simulink model "SHIP_DOWN_PT2000_matlab_2017"  (R2018b)
settings: Solver=ode8  StartTime=0.0  StopTime=2.5  RelTol=1e-3
undefined symbols (not defined in the file): Cout_c, Cout_r, Cvh_c, Cvh_r, dellay_f1, dellay_f2, dellay_f3, dellay_f4, dellay_f5, dellay_f6, DiscIntNeverNeededParam, f, L1_l, L1_r, Lvh_l, Lvh_r, R_out, Uout, Uvh
libraries: powerlib x92, simulink x18, simulink_extras x18, powerlib_meascontrol x13
(part 1 of 2)
settings Model: Creator=Anton  LastModifiedBy=VID Company
settings SFSimCC: SimUseLocalCustomCode=off
settings RTWCC: RTWUseLocalCustomCode=off
settings CodeAppCC: StateflowObjectComments=on
settings SimscapeCC: SimscapeNormalizeSystem=off

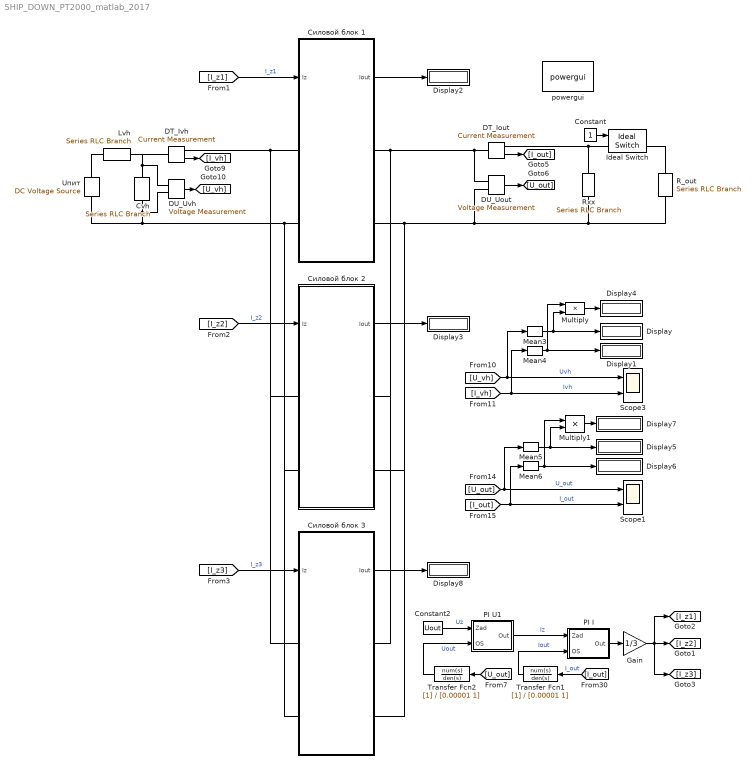
== system SHIP_DOWN_PT2000_matlab_2017 ==
  Constant : Constant
  Constant2 : Constant  Value=Uout
  Cvh : powerlib/Elements/Series RLC Branch  LConnTagsString=__new0  RConnTagsString=__new0  BranchType=RC  Resistance=Cvh_r  Inductance=1e-3  SetiL0=off  InitialCurrent=0  Capacitance=Cvh_c  Setx0=on  InitialVoltage=Uvh  Measurements=Branch voltage
      settings: SourceProductName=Simscape Electrical
  DT_Iout : powerlib/Measurements/Current Measurement  PhasorSimulation=off  OutputType=Complex  PSBequivalent=0
      settings: SourceProductName=Simscape Electrical
  DT_Ivh : powerlib/Measurements/Current Measurement  PhasorSimulation=off  OutputType=Complex  PSBequivalent=0
      settings: SourceProductName=Simscape Electrical
  DU_Uout : powerlib/Measurements/Voltage Measurement  PhasorSimulation=off  OutputType=Complex  PSBequivalent=0
      settings: SourceProductName=Simscape Electrical
  DU_Uvh : powerlib/Measurements/Voltage Measurement  PhasorSimulation=off  OutputType=Complex  PSBequivalent=0
      settings: SourceProductName=Simscape Electrical
  Display{,1..8} (9 alike) : Display
  Gain : Gain  Gain=1/3
  Ideal Switch : powerlib/Power Electronics/Ideal Switch  Ron=0.001  Lon=0  IC=0  Rs=1e5  Cs=inf  Measurements=on
  Lvh : powerlib/Elements/Series RLC Branch  LConnTagsString=__new0  RConnTagsString=__new0  BranchType=RL  Resistance=Lvh_r  Inductance=Lvh_l  SetiL0=off  InitialCurrent=0  Capacitance=1e-6  Setx0=off  InitialVoltage=0  Measurements=None
      settings: SourceProductName=Simscape Electrical
  Mean{3..6} (4 alike) : powerlib_meascontrol/Measurements/Mean  Freq=1000  Vinit=0  Ts=0
  Multiply : Product
  Multiply1 : Product
  PI I : Subsystem
  PI U1 : Subsystem
  R_out : powerlib/Elements/Series RLC Branch  LConnTagsString=__new0  RConnTagsString=__new0  BranchType=R  Resistance=R_out  Inductance=1e-3  SetiL0=off  InitialCurrent=0  Capacitance=1e-6  Setx0=off  InitialVoltage=0  Measurements=None
      settings: SourceProductName=Simscape Electrical
  Rxx : powerlib/Elements/Series RLC Branch  LConnTagsString=__new0  RConnTagsString=__new0  BranchType=R  Resistance=200  Inductance=1e-3  SetiL0=off  InitialCurrent=0  Capacitance=Cout_c  Setx0=on  InitialVoltage=0  Measurements=Branch voltage
      settings: SourceProductName=Simscape Electrical
  Scope1 : Scope  NumInputPorts=2
  Scope3 : Scope  NumInputPorts=2
  Transfer Fcn1 : TransferFcn  Denominator=[0.00001 1]
  Transfer Fcn2 : TransferFcn  Denominator=[0.00001 1]
  Uпит : powerlib/Electrical Sources/DC Voltage Source  Amplitude=Uvh  Measurements=None
      settings: SourceProductName=Simscape Electrical
  powergui : powerlib/powergui  Priority=1  SimulationMode=Discrete  SampleTime=1e-6  frequency=60  Iterations=50  frequencyindice=0  Pbase=100e6  ErrMax=1e-4  UnitsV=kV  UnitsW=MW  buscounter=0  FunctionMessages=off  echomessages=off  EnableUseOfTLC=off  CurrentSourceSwitches=off  DisableSnubberDevices=off  DisableRonSwitches=off  DisableVfSwitches=off  DisplayEquations=off  SolverType=Tustin/Backward Euler (TBE)  Interpol=off  ExternalGateDelay=off  methode=off  Ts=100  x0status=blocks  SPID=off  SwTol=0  HookPort=off  RestoreLinks=warning  ResistiveCurrentMeasurement=off  Frange=[0:2:500]  Ylog=off  Xlog=on  ShowGrid=off  save=off  variable=ZData  structure=0  ZoomFFT=off  StartTime=0.0  cycles=1  DisplayStyle=1  fundamental=60  FreqAxis=off  MaxFrequency=1000  frequencyindicesteady=1  RmsSteady=1  display=off
  Силовой блок 1 : Subsystem
  Силовой блок 2 : Subsystem
  Силовой блок 3 : Subsystem
  wires:
  Transfer Fcn2/1 -> PI U1/2(OS)  "Uout"
  PI U1/1(Out) -> PI I/1(Zad)  "Iz"
  Constant2/1 -> PI U1/1(Zad)  "Uz"
  DT_Iout/1 -> [I_out]
  DU_Uout/1 -> [U_out]
  [U_out] -> Transfer Fcn2/1
  DT_Ivh/1 -> [I_vh]
  DU_Uvh/1 -> [U_vh]
  [I_vh] -> Scope3/2, Mean4/1  "Ivh"
  [U_vh] -> Mean3/1, Scope3/1  "Uvh"
  Mean3/1 -> Display/1, Multiply/2
  Mean4/1 -> Display1/1, Multiply/1
  Multiply/1 -> Display4/1
  [U_out] -> Mean5/1, Scope1/1  "U_out"
  [I_out] -> Mean6/1, Scope1/2  "I_out"
  [I_out] -> Transfer Fcn1/1  "I_out"
  Transfer Fcn1/1 -> PI I/2(OS)  "Iout"
  PI I/1(Out) -> Gain/1
  Constant/1 -> Ideal Switch/1
  Gain/1 -> [I_z3], [I_z1], [I_z2]
  Силовой блок 1/1(Iout) -> Display2/1
  [I_z1] -> Силовой блок 1/1(Iz)  "I_z1"
  Multiply1/1 -> Display7/1
  Mean6/1 -> Display6/1, Multiply1/1
  Mean5/1 -> Display5/1, Multiply1/2
  [I_z2] -> Силовой блок 2/1(Iz)  "I_z2"
  [I_z3] -> Силовой блок 3/1(Iz)  "I_z3"
  Силовой блок 2/1(Iout) -> Display3/1
  Силовой блок 3/1(Iout) -> Display8/1
  connections:
  Cvh/RConn1 -- Силовой блок 3/LConn2 -- Силовой блок 2/LConn2 -- Силовой блок 1/LConn2 -- Uпит/LConn1 -- DU_Uvh/LConn2
  Lvh/LConn1 -- Uпит/RConn1
  Ideal Switch/RConn1 -- R_out/LConn1
  Силовой блок 3/RConn1 -- Силовой блок 2/RConn1 -- DU_Uout/LConn1 -- DT_Iout/LConn1 -- Силовой блок 1/RConn1
  DU_Uvh/LConn1 -- DT_Ivh/LConn1 -- Lvh/RConn1 -- Cvh/LConn1
  Rxx/RConn1 -- R_out/RConn1 -- Силовой блок 3/RConn2 -- Силовой блок 2/RConn2 -- Силовой блок 1/RConn2 -- DU_Uout/LConn2
  DT_Ivh/RConn1 -- Силовой блок 3/LConn1 -- Силовой блок 2/LConn1 -- Силовой блок 1/LConn1
  Ideal Switch/LConn1 -- DT_Iout/RConn1 -- Rxx/LConn1

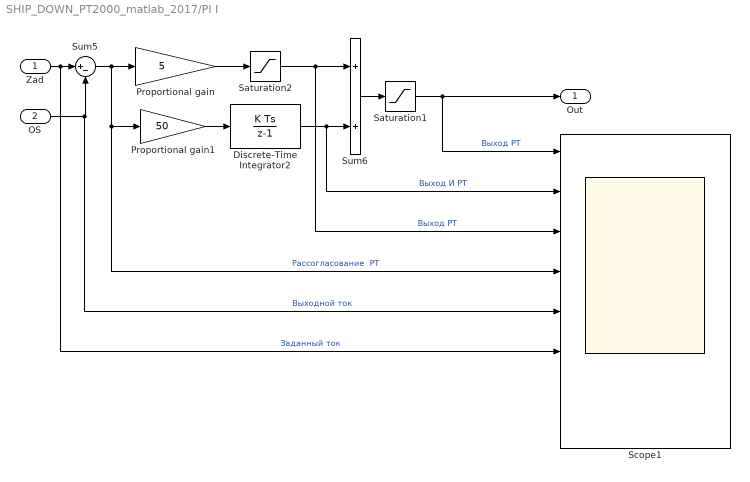
== system SHIP_DOWN_PT2000_matlab_2017/PI I ==
  Zad : Inport
  OS : Inport  Port=2
  Discrete-Time Integrator2 : DiscreteIntegrator  SampleTime=-1  LimitOutput=on  UpperSaturationLimit=1900  LowerSaturationLimit=0  ICPrevOutput=DiscIntNeverNeededParam  ICPrevScaledInput=DiscIntNeverNeededParam
  Proportional gain : Gain  Gain=5  SaturateOnIntegerOverflow=on  OutDataTypeStr=Inherit: Same as input  ParamDataTypeStr=Inherit: Same as input
  Proportional gain1 : Gain  Gain=50  SaturateOnIntegerOverflow=on  OutDataTypeStr=Inherit: Same as input  ParamDataTypeStr=Inherit: Same as input
  Saturation1 : Saturate  UpperLimit=1900  LowerLimit=0
  Saturation2 : Saturate  UpperLimit=1900  LowerLimit=0
  Scope1 : Scope  NumInputPorts=8
  Sum5 : Sum  Inputs=|+-  SaturateOnIntegerOverflow=on  InputSameDT=on  OutDataTypeStr=Inherit: Same as first input
  Sum6 : Sum  SaturateOnIntegerOverflow=on  InputSameDT=on  OutDataTypeStr=Inherit: Same as first input
  Out : Outport
  wires:
  Proportional gain/1 -> Saturation2/1
  Discrete-Time Integrator2/1 -> Sum6/2, Scope1/2  "Выход И РТ"
  OS/1 -> Scope1/5, Sum5/2  "Выходной ток"
  Zad/1 -> Scope1/6, Sum5/1  "Заданный ток"
  Sum5/1 -> Proportional gain1/1, Scope1/4, Proportional gain/1  "Рассогласование  РТ"
  Sum6/1 -> Saturation1/1
  Saturation1/1 -> Out/1, Scope1/1  "Выход РТ"
  Proportional gain1/1 -> Discrete-Time Integrator2/1
  Saturation2/1 -> Scope1/3, Sum6/1  "Выход РТ"

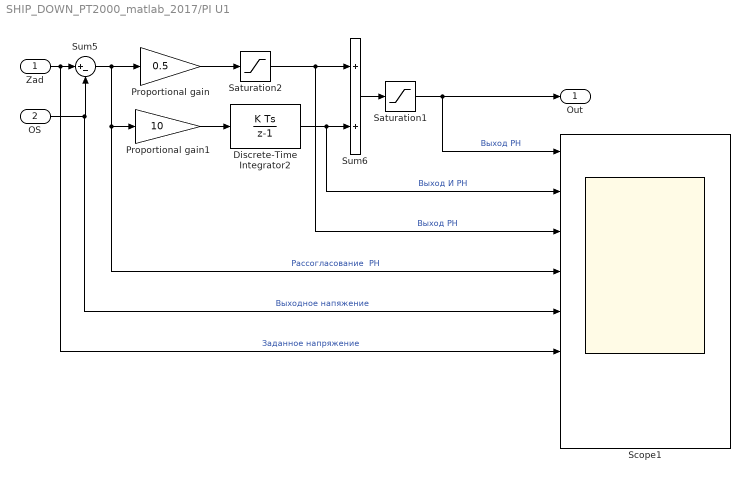
== system SHIP_DOWN_PT2000_matlab_2017/PI U1 ==
  Zad : Inport
  OS : Inport  Port=2
  Discrete-Time Integrator2 : DiscreteIntegrator  SampleTime=-1  LimitOutput=on  UpperSaturationLimit=1900  LowerSaturationLimit=0  ICPrevOutput=DiscIntNeverNeededParam  ICPrevScaledInput=DiscIntNeverNeededParam
  Proportional gain : Gain  Gain=0.5  SaturateOnIntegerOverflow=on  OutDataTypeStr=Inherit: Same as input  ParamDataTypeStr=Inherit: Same as input
  Proportional gain1 : Gain  Gain=10  SaturateOnIntegerOverflow=on  OutDataTypeStr=Inherit: Same as input  ParamDataTypeStr=Inherit: Same as input
  Saturation1 : Saturate  UpperLimit=1900  LowerLimit=0
  Saturation2 : Saturate  UpperLimit=1900  LowerLimit=0
  Scope1 : Scope  NumInputPorts=8
  Sum5 : Sum  Inputs=|+-  SaturateOnIntegerOverflow=on  InputSameDT=on  OutDataTypeStr=Inherit: Same as first input
  Sum6 : Sum  SaturateOnIntegerOverflow=on  InputSameDT=on  OutDataTypeStr=Inherit: Same as first input
  Out : Outport
  wires:
  Proportional gain/1 -> Saturation2/1
  Discrete-Time Integrator2/1 -> Sum6/2, Scope1/2  "Выход И РН"
  OS/1 -> Scope1/5, Sum5/2  "Выходное напяжение"
  Zad/1 -> Scope1/6, Sum5/1  "Заданное напряжение"
  Sum5/1 -> Proportional gain1/1, Scope1/4, Proportional gain/1  "Рассогласование  РН"
  Sum6/1 -> Saturation1/1
  Saturation1/1 -> Out/1, Scope1/1  "Выход РН"
  Proportional gain1/1 -> Discrete-Time Integrator2/1
  Saturation2/1 -> Scope1/3, Sum6/1  "Выход РН"

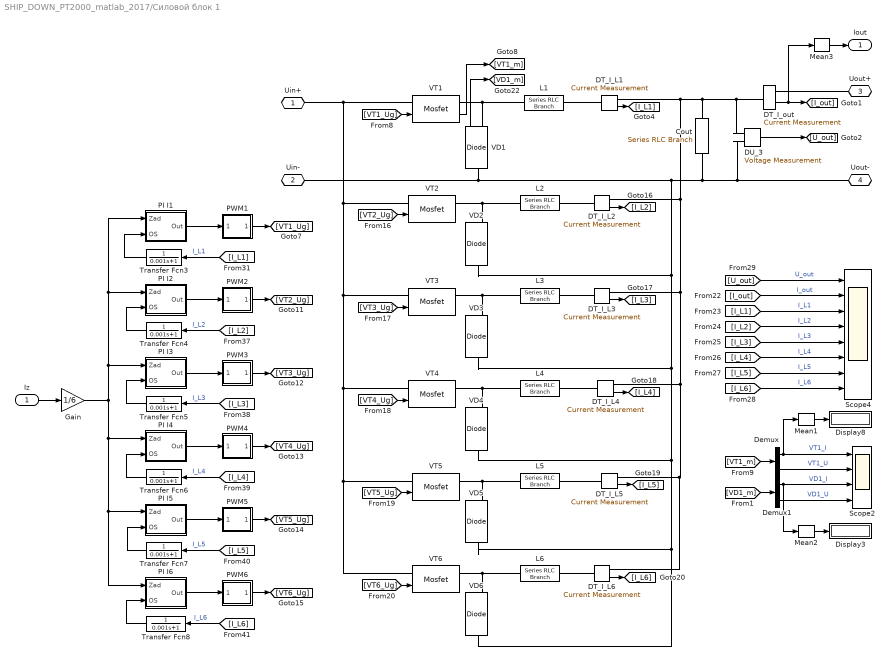
== system SHIP_DOWN_PT2000_matlab_2017/Силовой блок 1 ==
  Iz : Inport
  Cout : powerlib/Elements/Series RLC Branch  LConnTagsString=__new0  RConnTagsString=__new0  BranchType=RC  Resistance=Cout_r  Inductance=1e-3  SetiL0=off  InitialCurrent=0  Capacitance=Cout_c  Setx0=on  InitialVoltage=0  Measurements=Branch voltage
      settings: SourceProductName=Simscape Electrical
  DT_I_L{1..6} (6 alike) : powerlib/Measurements/Current Measurement  PhasorSimulation=off  OutputType=Complex  PSBequivalent=0
      settings: SourceProductName=Simscape Electrical
  DT_I_out : powerlib/Measurements/Current Measurement  PhasorSimulation=off  OutputType=Complex  PSBequivalent=0
      settings: SourceProductName=Simscape Electrical
  DU_3 : powerlib/Measurements/Voltage Measurement  PhasorSimulation=off  OutputType=Complex  PSBequivalent=0
      settings: SourceProductName=Simscape Electrical
  Demux : Demux  Outputs=2
  Demux1 : Demux  Outputs=2
  Display3 : Display
  Display8 : Display
  Gain : Gain  Gain=1/6
  L{1..6} (6 alike) : powerlib/Elements/Series RLC Branch  LConnTagsString=__new0  RConnTagsString=__new0  BranchType=RL  Resistance=L1_r  Inductance=L1_l  SetiL0=off  InitialCurrent=0  Capacitance=1e-6  Setx0=off  InitialVoltage=0  Measurements=None
      settings: SourceProductName=Simscape Electrical
  Mean1 : powerlib_meascontrol/Measurements/Mean  Freq=4000  Vinit=0  Ts=0
  Mean2 : powerlib_meascontrol/Measurements/Mean  Freq=4000  Vinit=0  Ts=0
  Mean3 : powerlib_meascontrol/Measurements/Mean  Freq=4000  Vinit=0  Ts=0
  PI I1 : Subsystem
  PI I2 : Subsystem
  PI I3 : Subsystem
  PI I4 : Subsystem
  PI I5 : Subsystem
  PI I6 : Subsystem
  PWM1 : Subsystem
  PWM2 : Subsystem
  PWM3 : Subsystem
  PWM4 : Subsystem
  PWM5 : Subsystem
  PWM6 : Subsystem
  Scope2 : Scope  NumInputPorts=4
  Scope4 : Scope  NumInputPorts=8
  Transfer Fcn{3..8} (6 alike) : TransferFcn  Denominator=[0.001 1]
  VD{1..6} (6 alike) : powerlib/Power Electronics/Diode  Ron=0.001  Lon=0  Vf=1  IC=0  UseSnubber=off  Rs=inf  Cs=inf  Measurements=on
      settings: SourceProductName=Simscape Electrical
  VT{1..6} (6 alike) : powerlib/Power Electronics/Mosfet  Ron=10e-3  Lon=inf  Rd=3e-3  Vfd=1  IC=0  Rs=1e5  Cs=inf  Measurements=on
      settings: SourceProductName=Simscape Electrical
  Uin+ : PMIOPort  Side=Left
  Uin- : PMIOPort  Port=2  Side=Left
  Uout+ : PMIOPort  Port=3  Side=Right
  Uout- : PMIOPort  Port=4  Side=Right
  Iout : Outport
  wires:
  DT_I_L1/1 -> [I_L1]
  VD1/1 -> [VD1_m]
  [VT4_Ug] -> VT4/1
  VT1/1 -> [VT1_m]
  DT_I_L6/1 -> [I_L6]
  DT_I_L5/1 -> [I_L5]
  [VT1_Ug] -> VT1/1
  [VT5_Ug] -> VT5/1
  [VT6_Ug] -> VT6/1
  DT_I_L4/1 -> [I_L4]
  DT_I_L2/1 -> [I_L2]
  DT_I_L3/1 -> [I_L3]
  [VT3_Ug] -> VT3/1
  [VT2_Ug] -> VT2/1
  PI I5/1(Out) -> PWM5/1(Uz)
  PI I2/1(Out) -> PWM2/1(Uz)
  PI I3/1(Out) -> PWM3/1(Uz)
  Transfer Fcn7/1 -> PI I5/2(OS)
  [I_L5] -> Transfer Fcn7/1  "I_L5"
  [I_L3] -> Transfer Fcn5/1  "I_L3"
  PWM3/1(CH1) -> [VT3_Ug]
  Transfer Fcn8/1 -> PI I6/2(OS)
  Transfer Fcn3/1 -> PI I1/2(OS)
  Iz/1 -> Gain/1
  Transfer Fcn4/1 -> PI I2/2(OS)
  [I_L2] -> Transfer Fcn4/1  "I_L2"
  [I_L4] -> Transfer Fcn6/1  "I_L4"
  PI I1/1(Out) -> PWM1/1(Uz)
  Transfer Fcn5/1 -> PI I3/2(OS)
  PWM5/1(CH1) -> [VT5_Ug]
  PWM2/1(CH1) -> [VT2_Ug]
  PWM1/1(CH1) -> [VT1_Ug]
  PWM4/1(CH1) -> [VT4_Ug]
  [I_L6] -> Transfer Fcn8/1  "I_L6"
  [I_L1] -> Transfer Fcn3/1  "I_L1"
  PI I4/1(Out) -> PWM4/1(Uz)
  Transfer Fcn6/1 -> PI I4/2(OS)
  PI I6/1(Out) -> PWM6/1(Uz)
  PWM6/1(CH1) -> [VT6_Ug]
  Demux/1 -> Scope2/1, Mean1/1  "VT1_I"
  Demux1/2 -> Scope2/4  "VD1_U"
  Demux1/1 -> Mean2/1, Scope2/3  "VD1_I"
  Mean1/1 -> Display8/1
  Mean2/1 -> Display3/1
  [VD1_m] -> Demux1/1
  [VT1_m] -> Demux/1
  Demux/2 -> Scope2/2  "VT1_U"
  [I_out] -> Scope4/2  "I_out"
  [U_out] -> Scope4/1  "U_out"
  [I_L2] -> Scope4/4  "I_L2"
  [I_L4] -> Scope4/6  "I_L4"
  [I_L3] -> Scope4/5  "I_L3"
  [I_L6] -> Scope4/8  "I_L6"
  [I_L1] -> Scope4/3  "I_L1"
  [I_L5] -> Scope4/7  "I_L5"
  Gain/1 -> PI I4/1(Zad), PI I6/1(Zad), PI I5/1(Zad), PI I3/1(Zad), PI I1/1(Zad), PI I2/1(Zad)
  DT_I_out/1 -> Mean3/1, [I_out]
  DU_3/1 -> [U_out]
  Mean3/1 -> Iout/1
  connections:
  VD5/RConn1 -- L5/LConn1 -- VT5/RConn1
  VD1/LConn1 -- DU_3/LConn2 -- Uout-/RConn1 -- Cout/RConn1 -- VD6/LConn1 -- VD5/LConn1 -- VD4/LConn1 -- VD3/LConn1 -- VD2/LConn1 -- Uin-/RConn1
  VD6/RConn1 -- L6/LConn1 -- VT6/RConn1
  VD1/RConn1 -- VT1/RConn1 -- L1/LConn1
  VD3/RConn1 -- L3/LConn1 -- VT3/RConn1
  L2/LConn1 -- VD2/RConn1 -- VT2/RConn1
  VD4/RConn1 -- L4/LConn1 -- VT4/RConn1
  DT_I_L5/LConn1 -- L5/RConn1
  DT_I_L3/LConn1 -- L3/RConn1
  DT_I_L4/LConn1 -- L4/RConn1
  DT_I_L1/LConn1 -- L1/RConn1
  L2/RConn1 -- DT_I_L2/LConn1
  L6/RConn1 -- DT_I_L6/LConn1
  Uin+/RConn1 -- VT6/LConn1 -- VT5/LConn1 -- VT4/LConn1 -- VT3/LConn1 -- VT2/LConn1 -- VT1/LConn1
  DT_I_L1/RConn1 -- DU_3/LConn1 -- DT_I_out/LConn1 -- Cout/LConn1 -- DT_I_L6/RConn1 -- DT_I_L5/RConn1 -- DT_I_L4/RConn1 -- DT_I_L3/RConn1 -- DT_I_L2/RConn1
  DT_I_out/RConn1 -- Uout+/RConn1

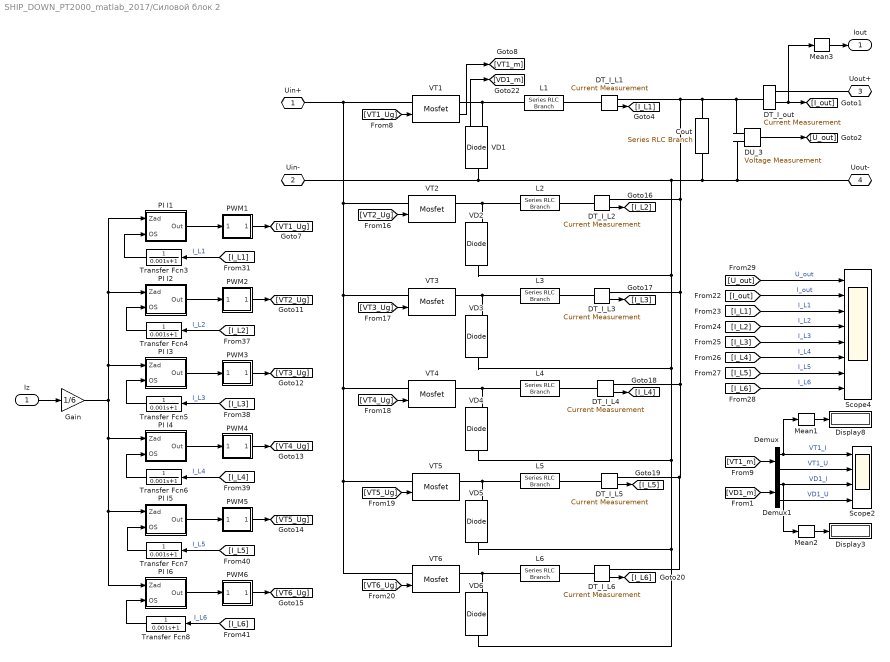
== system SHIP_DOWN_PT2000_matlab_2017/Силовой блок 2 ==
  Iz : Inport
  Cout : powerlib/Elements/Series RLC Branch  LConnTagsString=__new0  RConnTagsString=__new0  BranchType=RC  Resistance=Cout_r  Inductance=1e-3  SetiL0=off  InitialCurrent=0  Capacitance=Cout_c  Setx0=on  InitialVoltage=0  Measurements=Branch voltage
      settings: SourceProductName=Simscape Electrical
  DT_I_L{1..6} (6 alike) : powerlib/Measurements/Current Measurement  PhasorSimulation=off  OutputType=Complex  PSBequivalent=0
      settings: SourceProductName=Simscape Electrical
  DT_I_out : powerlib/Measurements/Current Measurement  PhasorSimulation=off  OutputType=Complex  PSBequivalent=0
      settings: SourceProductName=Simscape Electrical
  DU_3 : powerlib/Measurements/Voltage Measurement  PhasorSimulation=off  OutputType=Complex  PSBequivalent=0
      settings: SourceProductName=Simscape Electrical
  Demux : Demux  Outputs=2
  Demux1 : Demux  Outputs=2
  Display3 : Display
  Display8 : Display
  Gain : Gain  Gain=1/6
  L{1..6} (6 alike) : powerlib/Elements/Series RLC Branch  LConnTagsString=__new0  RConnTagsString=__new0  BranchType=RL  Resistance=L1_r  Inductance=L1_l  SetiL0=off  InitialCurrent=0  Capacitance=1e-6  Setx0=off  InitialVoltage=0  Measurements=None
      settings: SourceProductName=Simscape Electrical
  Mean1 : powerlib_meascontrol/Measurements/Mean  Freq=4000  Vinit=0  Ts=0
  Mean2 : powerlib_meascontrol/Measurements/Mean  Freq=4000  Vinit=0  Ts=0
  Mean3 : powerlib_meascontrol/Measurements/Mean  Freq=4000  Vinit=0  Ts=0
  PI I1 : Subsystem
  PI I2 : Subsystem
  PI I3 : Subsystem
  PI I4 : Subsystem
  PI I5 : Subsystem
  PI I6 : Subsystem
  PWM1 : Subsystem
  PWM2 : Subsystem
  PWM3 : Subsystem
  PWM4 : Subsystem
  PWM5 : Subsystem
  PWM6 : Subsystem
  Scope2 : Scope  NumInputPorts=4
  Scope4 : Scope  NumInputPorts=8
  Transfer Fcn{3..8} (6 alike) : TransferFcn  Denominator=[0.001 1]
  VD{1..6} (6 alike) : powerlib/Power Electronics/Diode  Ron=0.001  Lon=0  Vf=1  IC=0  UseSnubber=off  Rs=inf  Cs=inf  Measurements=on
      settings: SourceProductName=Simscape Electrical
  VT{1..6} (6 alike) : powerlib/Power Electronics/Mosfet  Ron=10e-3  Lon=inf  Rd=3e-3  Vfd=1  IC=0  Rs=1e5  Cs=inf  Measurements=on
      settings: SourceProductName=Simscape Electrical
  Uin+ : PMIOPort  Side=Left
  Uin- : PMIOPort  Port=2  Side=Left
  Uout+ : PMIOPort  Port=3  Side=Right
  Uout- : PMIOPort  Port=4  Side=Right
  Iout : Outport
  wires:
  DT_I_L1/1 -> [I_L1]
  VD1/1 -> [VD1_m]
  [VT4_Ug] -> VT4/1
  VT1/1 -> [VT1_m]
  DT_I_L6/1 -> [I_L6]
  DT_I_L5/1 -> [I_L5]
  [VT1_Ug] -> VT1/1
  [VT5_Ug] -> VT5/1
  [VT6_Ug] -> VT6/1
  DT_I_L4/1 -> [I_L4]
  DT_I_L2/1 -> [I_L2]
  DT_I_L3/1 -> [I_L3]
  [VT3_Ug] -> VT3/1
  [VT2_Ug] -> VT2/1
  PI I5/1(Out) -> PWM5/1(Uz)
  PI I2/1(Out) -> PWM2/1(Uz)
  PI I3/1(Out) -> PWM3/1(Uz)
  Transfer Fcn7/1 -> PI I5/2(OS)
  [I_L5] -> Transfer Fcn7/1  "I_L5"
  [I_L3] -> Transfer Fcn5/1  "I_L3"
  PWM3/1(CH1) -> [VT3_Ug]
  Transfer Fcn8/1 -> PI I6/2(OS)
  Transfer Fcn3/1 -> PI I1/2(OS)
  Iz/1 -> Gain/1
  Transfer Fcn4/1 -> PI I2/2(OS)
  [I_L2] -> Transfer Fcn4/1  "I_L2"
  [I_L4] -> Transfer Fcn6/1  "I_L4"
  PI I1/1(Out) -> PWM1/1(Uz)
  Transfer Fcn5/1 -> PI I3/2(OS)
  PWM5/1(CH1) -> [VT5_Ug]
  PWM2/1(CH1) -> [VT2_Ug]
  PWM1/1(CH1) -> [VT1_Ug]
  PWM4/1(CH1) -> [VT4_Ug]
  [I_L6] -> Transfer Fcn8/1  "I_L6"
  [I_L1] -> Transfer Fcn3/1  "I_L1"
  PI I4/1(Out) -> PWM4/1(Uz)
  Transfer Fcn6/1 -> PI I4/2(OS)
  PI I6/1(Out) -> PWM6/1(Uz)
  PWM6/1(CH1) -> [VT6_Ug]
  Demux/1 -> Scope2/1, Mean1/1  "VT1_I"
  Demux1/2 -> Scope2/4  "VD1_U"
  Demux1/1 -> Mean2/1, Scope2/3  "VD1_I"
  Mean1/1 -> Display8/1
  Mean2/1 -> Display3/1
  [VD1_m] -> Demux1/1
  [VT1_m] -> Demux/1
  Demux/2 -> Scope2/2  "VT1_U"
  [I_out] -> Scope4/2  "I_out"
  [U_out] -> Scope4/1  "U_out"
  [I_L2] -> Scope4/4  "I_L2"
  [I_L4] -> Scope4/6  "I_L4"
  [I_L3] -> Scope4/5  "I_L3"
  [I_L6] -> Scope4/8  "I_L6"
  [I_L1] -> Scope4/3  "I_L1"
  [I_L5] -> Scope4/7  "I_L5"
  Gain/1 -> PI I4/1(Zad), PI I6/1(Zad), PI I5/1(Zad), PI I3/1(Zad), PI I1/1(Zad), PI I2/1(Zad)
  DT_I_out/1 -> Mean3/1, [I_out]
  DU_3/1 -> [U_out]
  Mean3/1 -> Iout/1
  connections:
  VD5/RConn1 -- L5/LConn1 -- VT5/RConn1
  VD6/LConn1 -- VD5/LConn1 -- VD4/LConn1 -- VD3/LConn1 -- VD2/LConn1 -- VD1/LConn1 -- Uin-/RConn1 -- DU_3/LConn2 -- Uout-/RConn1 -- Cout/RConn1
  VD6/RConn1 -- L6/LConn1 -- VT6/RConn1
  VD1/RConn1 -- VT1/RConn1 -- L1/LConn1
  VD3/RConn1 -- L3/LConn1 -- VT3/RConn1
  L2/LConn1 -- VD2/RConn1 -- VT2/RConn1
  VD4/RConn1 -- L4/LConn1 -- VT4/RConn1
  DT_I_L5/LConn1 -- L5/RConn1
  DT_I_L3/LConn1 -- L3/RConn1
  DT_I_L4/LConn1 -- L4/RConn1
  DT_I_L1/LConn1 -- L1/RConn1
  L2/RConn1 -- DT_I_L2/LConn1
  L6/RConn1 -- DT_I_L6/LConn1
  Uin+/RConn1 -- VT6/LConn1 -- VT5/LConn1 -- VT4/LConn1 -- VT3/LConn1 -- VT2/LConn1 -- VT1/LConn1
  DU_3/LConn1 -- DT_I_out/LConn1 -- Cout/LConn1 -- DT_I_L1/RConn1 -- DT_I_L6/RConn1 -- DT_I_L5/RConn1 -- DT_I_L4/RConn1 -- DT_I_L3/RConn1 -- DT_I_L2/RConn1
  DT_I_out/RConn1 -- Uout+/RConn1

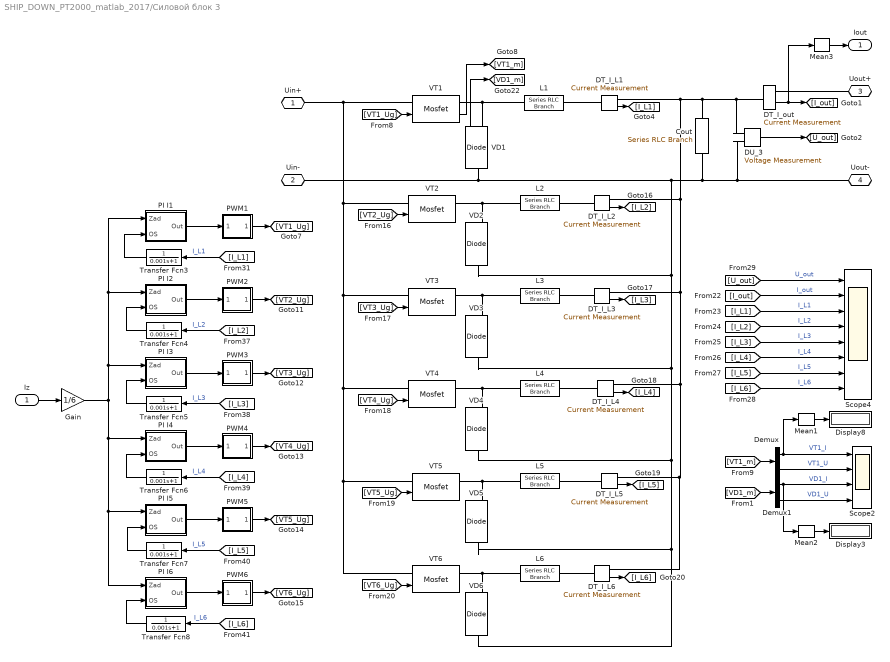
== system SHIP_DOWN_PT2000_matlab_2017/Силовой блок 3 ==
  Iz : Inport
  Cout : powerlib/Elements/Series RLC Branch  LConnTagsString=__new0  RConnTagsString=__new0  BranchType=RC  Resistance=Cout_r  Inductance=1e-3  SetiL0=off  InitialCurrent=0  Capacitance=Cout_c  Setx0=on  InitialVoltage=0  Measurements=Branch voltage
      settings: SourceProductName=Simscape Electrical
  DT_I_L{1..6} (6 alike) : powerlib/Measurements/Current Measurement  PhasorSimulation=off  OutputType=Complex  PSBequivalent=0
      settings: SourceProductName=Simscape Electrical
  DT_I_out : powerlib/Measurements/Current Measurement  PhasorSimulation=off  OutputType=Complex  PSBequivalent=0
      settings: SourceProductName=Simscape Electrical
  DU_3 : powerlib/Measurements/Voltage Measurement  PhasorSimulation=off  OutputType=Complex  PSBequivalent=0
      settings: SourceProductName=Simscape Electrical
  Demux : Demux  Outputs=2
  Demux1 : Demux  Outputs=2
  Display3 : Display
  Display8 : Display
  Gain : Gain  Gain=1/6
  L{1..6} (6 alike) : powerlib/Elements/Series RLC Branch  LConnTagsString=__new0  RConnTagsString=__new0  BranchType=RL  Resistance=L1_r  Inductance=L1_l  SetiL0=off  InitialCurrent=0  Capacitance=1e-6  Setx0=off  InitialVoltage=0  Measurements=None
      settings: SourceProductName=Simscape Electrical
  Mean1 : powerlib_meascontrol/Measurements/Mean  Freq=4000  Vinit=0  Ts=0
  Mean2 : powerlib_meascontrol/Measurements/Mean  Freq=4000  Vinit=0  Ts=0
  Mean3 : powerlib_meascontrol/Measurements/Mean  Freq=4000  Vinit=0  Ts=0
  PI I1 : Subsystem
  PI I2 : Subsystem
  PI I3 : Subsystem
  PI I4 : Subsystem
  PI I5 : Subsystem
  PI I6 : Subsystem
  PWM1 : Subsystem
  PWM2 : Subsystem
  PWM3 : Subsystem
  PWM4 : Subsystem
  PWM5 : Subsystem
  PWM6 : Subsystem
  Scope2 : Scope  NumInputPorts=4
  Scope4 : Scope  NumInputPorts=8
  Transfer Fcn{3..8} (6 alike) : TransferFcn  Denominator=[0.001 1]
  VD{1..6} (6 alike) : powerlib/Power Electronics/Diode  Ron=0.001  Lon=0  Vf=1  IC=0  UseSnubber=off  Rs=inf  Cs=inf  Measurements=on
      settings: SourceProductName=Simscape Electrical
  VT{1..6} (6 alike) : powerlib/Power Electronics/Mosfet  Ron=10e-3  Lon=inf  Rd=3e-3  Vfd=1  IC=0  Rs=1e5  Cs=inf  Measurements=on
      settings: SourceProductName=Simscape Electrical
  Uin+ : PMIOPort  Side=Left
  Uin- : PMIOPort  Port=2  Side=Left
  Uout+ : PMIOPort  Port=3  Side=Right
  Uout- : PMIOPort  Port=4  Side=Right
  Iout : Outport
  wires:
  DT_I_L1/1 -> [I_L1]
  VD1/1 -> [VD1_m]
  [VT4_Ug] -> VT4/1
  VT1/1 -> [VT1_m]
  DT_I_L6/1 -> [I_L6]
  DT_I_L5/1 -> [I_L5]
  [VT1_Ug] -> VT1/1
  [VT5_Ug] -> VT5/1
  [VT6_Ug] -> VT6/1
  DT_I_L4/1 -> [I_L4]
  DT_I_L2/1 -> [I_L2]
  DT_I_L3/1 -> [I_L3]
  [VT3_Ug] -> VT3/1
  [VT2_Ug] -> VT2/1
  PI I5/1(Out) -> PWM5/1(Uz)
  PI I2/1(Out) -> PWM2/1(Uz)
  PI I3/1(Out) -> PWM3/1(Uz)
  Transfer Fcn7/1 -> PI I5/2(OS)
  [I_L5] -> Transfer Fcn7/1  "I_L5"
  [I_L3] -> Transfer Fcn5/1  "I_L3"
  PWM3/1(CH1) -> [VT3_Ug]
  Transfer Fcn8/1 -> PI I6/2(OS)
  Transfer Fcn3/1 -> PI I1/2(OS)
  Iz/1 -> Gain/1
  Transfer Fcn4/1 -> PI I2/2(OS)
  [I_L2] -> Transfer Fcn4/1  "I_L2"
  [I_L4] -> Transfer Fcn6/1  "I_L4"
  PI I1/1(Out) -> PWM1/1(Uz)
  Transfer Fcn5/1 -> PI I3/2(OS)
  PWM5/1(CH1) -> [VT5_Ug]
  PWM2/1(CH1) -> [VT2_Ug]
  PWM1/1(CH1) -> [VT1_Ug]
  PWM4/1(CH1) -> [VT4_Ug]
  [I_L6] -> Transfer Fcn8/1  "I_L6"
  [I_L1] -> Transfer Fcn3/1  "I_L1"
  PI I4/1(Out) -> PWM4/1(Uz)
  Transfer Fcn6/1 -> PI I4/2(OS)
  PI I6/1(Out) -> PWM6/1(Uz)
  PWM6/1(CH1) -> [VT6_Ug]
  Demux/1 -> Scope2/1, Mean1/1  "VT1_I"
  Demux1/2 -> Scope2/4  "VD1_U"
  Demux1/1 -> Mean2/1, Scope2/3  "VD1_I"
  Mean1/1 -> Display8/1
  Mean2/1 -> Display3/1
  [VD1_m] -> Demux1/1
  [VT1_m] -> Demux/1
  Demux/2 -> Scope2/2  "VT1_U"
  [I_out] -> Scope4/2  "I_out"
  [U_out] -> Scope4/1  "U_out"
  [I_L2] -> Scope4/4  "I_L2"
  [I_L4] -> Scope4/6  "I_L4"
  [I_L3] -> Scope4/5  "I_L3"
  [I_L6] -> Scope4/8  "I_L6"
  [I_L1] -> Scope4/3  "I_L1"
  [I_L5] -> Scope4/7  "I_L5"
  Gain/1 -> PI I4/1(Zad), PI I6/1(Zad), PI I5/1(Zad), PI I3/1(Zad), PI I1/1(Zad), PI I2/1(Zad)
  DT_I_out/1 -> Mean3/1, [I_out]
  DU_3/1 -> [U_out]
  Mean3/1 -> Iout/1
  connections:
  VD5/RConn1 -- L5/LConn1 -- VT5/RConn1
  VD6/LConn1 -- VD5/LConn1 -- VD4/LConn1 -- VD3/LConn1 -- VD2/LConn1 -- VD1/LConn1 -- Uin-/RConn1 -- DU_3/LConn2 -- Uout-/RConn1 -- Cout/RConn1
  VD6/RConn1 -- L6/LConn1 -- VT6/RConn1
  VD1/RConn1 -- VT1/RConn1 -- L1/LConn1
  VD3/RConn1 -- L3/LConn1 -- VT3/RConn1
  L2/LConn1 -- VD2/RConn1 -- VT2/RConn1
  VD4/RConn1 -- L4/LConn1 -- VT4/RConn1
  DT_I_L5/LConn1 -- L5/RConn1
  DT_I_L3/LConn1 -- L3/RConn1
  DT_I_L4/LConn1 -- L4/RConn1
  DT_I_L1/LConn1 -- L1/RConn1
  L2/RConn1 -- DT_I_L2/LConn1
  L6/RConn1 -- DT_I_L6/LConn1
  Uin+/RConn1 -- VT6/LConn1 -- VT5/LConn1 -- VT4/LConn1 -- VT3/LConn1 -- VT2/LConn1 -- VT1/LConn1
  DU_3/LConn1 -- DT_I_out/LConn1 -- Cout/LConn1 -- DT_I_L1/RConn1 -- DT_I_L6/RConn1 -- DT_I_L5/RConn1 -- DT_I_L4/RConn1 -- DT_I_L3/RConn1 -- DT_I_L2/RConn1
  DT_I_out/RConn1 -- Uout+/RConn1

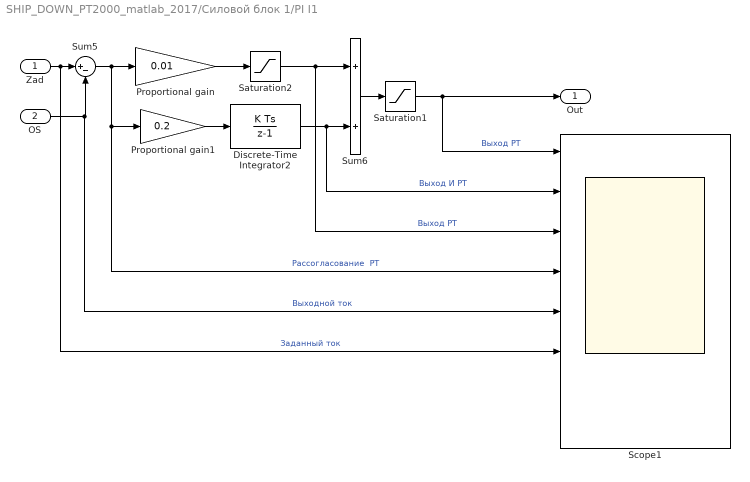
== system SHIP_DOWN_PT2000_matlab_2017/Силовой блок 1/PI I1 ==
  Zad : Inport
  OS : Inport  Port=2
  Discrete-Time Integrator2 : DiscreteIntegrator  SampleTime=-1  LimitOutput=on  UpperSaturationLimit=0.7  LowerSaturationLimit=0  ICPrevOutput=DiscIntNeverNeededParam  ICPrevScaledInput=DiscIntNeverNeededParam
  Proportional gain : Gain  Gain=0.01  SaturateOnIntegerOverflow=on  OutDataTypeStr=Inherit: Same as input  ParamDataTypeStr=Inherit: Same as input
  Proportional gain1 : Gain  Gain=0.2  SaturateOnIntegerOverflow=on  OutDataTypeStr=Inherit: Same as input  ParamDataTypeStr=Inherit: Same as input
  Saturation1 : Saturate  UpperLimit=0.7  LowerLimit=0
  Saturation2 : Saturate  UpperLimit=0.4  LowerLimit=0
  Scope1 : Scope  NumInputPorts=8
  Sum5 : Sum  Inputs=|+-  SaturateOnIntegerOverflow=on  InputSameDT=on  OutDataTypeStr=Inherit: Same as first input
  Sum6 : Sum  SaturateOnIntegerOverflow=on  InputSameDT=on  OutDataTypeStr=Inherit: Same as first input
  Out : Outport
  wires:
  Proportional gain/1 -> Saturation2/1
  Discrete-Time Integrator2/1 -> Sum6/2, Scope1/2  "Выход И РТ"
  OS/1 -> Scope1/5, Sum5/2  "Выходной ток"
  Zad/1 -> Scope1/6, Sum5/1  "Заданный ток"
  Sum5/1 -> Proportional gain1/1, Scope1/4, Proportional gain/1  "Рассогласование  РТ"
  Sum6/1 -> Saturation1/1
  Saturation1/1 -> Out/1, Scope1/1  "Выход РТ"
  Proportional gain1/1 -> Discrete-Time Integrator2/1
  Saturation2/1 -> Scope1/3, Sum6/1  "Выход РТ"

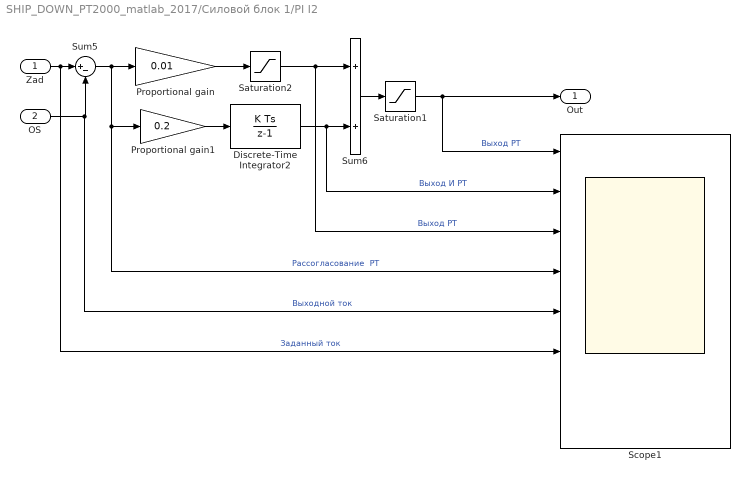
== system SHIP_DOWN_PT2000_matlab_2017/Силовой блок 1/PI I2 ==
  Zad : Inport
  OS : Inport  Port=2
  Discrete-Time Integrator2 : DiscreteIntegrator  SampleTime=-1  LimitOutput=on  UpperSaturationLimit=0.7  LowerSaturationLimit=0  ICPrevOutput=DiscIntNeverNeededParam  ICPrevScaledInput=DiscIntNeverNeededParam
  Proportional gain : Gain  Gain=0.01  SaturateOnIntegerOverflow=on  OutDataTypeStr=Inherit: Same as input  ParamDataTypeStr=Inherit: Same as input
  Proportional gain1 : Gain  Gain=0.2  SaturateOnIntegerOverflow=on  OutDataTypeStr=Inherit: Same as input  ParamDataTypeStr=Inherit: Same as input
  Saturation1 : Saturate  UpperLimit=0.7  LowerLimit=0
  Saturation2 : Saturate  UpperLimit=0.4  LowerLimit=0
  Scope1 : Scope  NumInputPorts=8
  Sum5 : Sum  Inputs=|+-  SaturateOnIntegerOverflow=on  InputSameDT=on  OutDataTypeStr=Inherit: Same as first input
  Sum6 : Sum  SaturateOnIntegerOverflow=on  InputSameDT=on  OutDataTypeStr=Inherit: Same as first input
  Out : Outport
  wires:
  Proportional gain/1 -> Saturation2/1
  Discrete-Time Integrator2/1 -> Sum6/2, Scope1/2  "Выход И РТ"
  OS/1 -> Scope1/5, Sum5/2  "Выходной ток"
  Zad/1 -> Scope1/6, Sum5/1  "Заданный ток"
  Sum5/1 -> Proportional gain1/1, Scope1/4, Proportional gain/1  "Рассогласование  РТ"
  Sum6/1 -> Saturation1/1
  Saturation1/1 -> Out/1, Scope1/1  "Выход РТ"
  Proportional gain1/1 -> Discrete-Time Integrator2/1
  Saturation2/1 -> Scope1/3, Sum6/1  "Выход РТ"

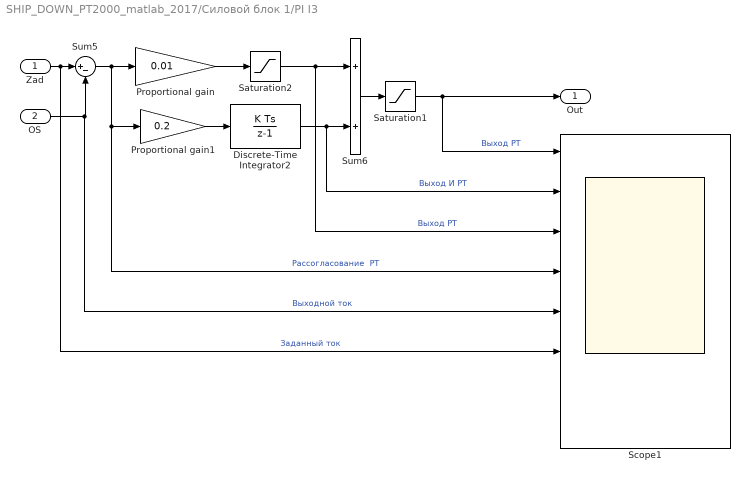
== system SHIP_DOWN_PT2000_matlab_2017/Силовой блок 1/PI I3 ==
  Zad : Inport
  OS : Inport  Port=2
  Discrete-Time Integrator2 : DiscreteIntegrator  SampleTime=-1  LimitOutput=on  UpperSaturationLimit=0.7  LowerSaturationLimit=0  ICPrevOutput=DiscIntNeverNeededParam  ICPrevScaledInput=DiscIntNeverNeededParam
  Proportional gain : Gain  Gain=0.01  SaturateOnIntegerOverflow=on  OutDataTypeStr=Inherit: Same as input  ParamDataTypeStr=Inherit: Same as input
  Proportional gain1 : Gain  Gain=0.2  SaturateOnIntegerOverflow=on  OutDataTypeStr=Inherit: Same as input  ParamDataTypeStr=Inherit: Same as input
  Saturation1 : Saturate  UpperLimit=0.7  LowerLimit=0
  Saturation2 : Saturate  UpperLimit=0.4  LowerLimit=0
  Scope1 : Scope  NumInputPorts=8
  Sum5 : Sum  Inputs=|+-  SaturateOnIntegerOverflow=on  InputSameDT=on  OutDataTypeStr=Inherit: Same as first input
  Sum6 : Sum  SaturateOnIntegerOverflow=on  InputSameDT=on  OutDataTypeStr=Inherit: Same as first input
  Out : Outport
  wires:
  Proportional gain/1 -> Saturation2/1
  Discrete-Time Integrator2/1 -> Sum6/2, Scope1/2  "Выход И РТ"
  OS/1 -> Scope1/5, Sum5/2  "Выходной ток"
  Zad/1 -> Scope1/6, Sum5/1  "Заданный ток"
  Sum5/1 -> Proportional gain1/1, Scope1/4, Proportional gain/1  "Рассогласование  РТ"
  Sum6/1 -> Saturation1/1
  Saturation1/1 -> Out/1, Scope1/1  "Выход РТ"
  Proportional gain1/1 -> Discrete-Time Integrator2/1
  Saturation2/1 -> Scope1/3, Sum6/1  "Выход РТ"

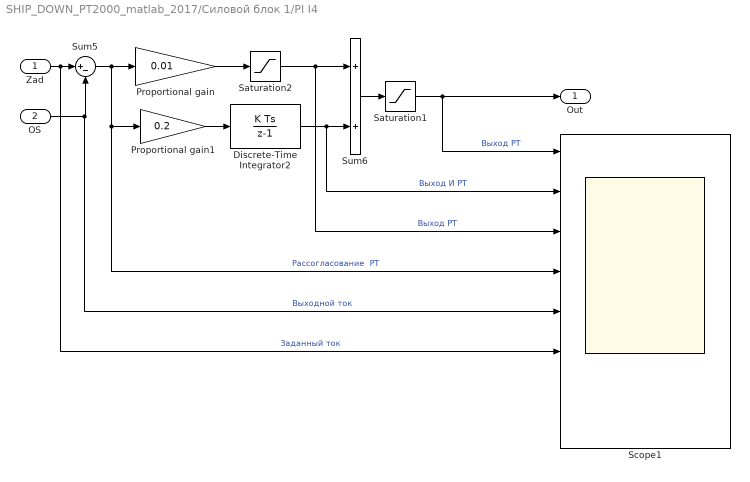
== system SHIP_DOWN_PT2000_matlab_2017/Силовой блок 1/PI I4 ==
  Zad : Inport
  OS : Inport  Port=2
  Discrete-Time Integrator2 : DiscreteIntegrator  SampleTime=-1  LimitOutput=on  UpperSaturationLimit=0.7  LowerSaturationLimit=0  ICPrevOutput=DiscIntNeverNeededParam  ICPrevScaledInput=DiscIntNeverNeededParam
  Proportional gain : Gain  Gain=0.01  SaturateOnIntegerOverflow=on  OutDataTypeStr=Inherit: Same as input  ParamDataTypeStr=Inherit: Same as input
  Proportional gain1 : Gain  Gain=0.2  SaturateOnIntegerOverflow=on  OutDataTypeStr=Inherit: Same as input  ParamDataTypeStr=Inherit: Same as input
  Saturation1 : Saturate  UpperLimit=0.7  LowerLimit=0
  Saturation2 : Saturate  UpperLimit=0.4  LowerLimit=0
  Scope1 : Scope  NumInputPorts=8
  Sum5 : Sum  Inputs=|+-  SaturateOnIntegerOverflow=on  InputSameDT=on  OutDataTypeStr=Inherit: Same as first input
  Sum6 : Sum  SaturateOnIntegerOverflow=on  InputSameDT=on  OutDataTypeStr=Inherit: Same as first input
  Out : Outport
  wires:
  Proportional gain/1 -> Saturation2/1
  Discrete-Time Integrator2/1 -> Sum6/2, Scope1/2  "Выход И РТ"
  OS/1 -> Scope1/5, Sum5/2  "Выходной ток"
  Zad/1 -> Scope1/6, Sum5/1  "Заданный ток"
  Sum5/1 -> Proportional gain1/1, Scope1/4, Proportional gain/1  "Рассогласование  РТ"
  Sum6/1 -> Saturation1/1
  Saturation1/1 -> Out/1, Scope1/1  "Выход РТ"
  Proportional gain1/1 -> Discrete-Time Integrator2/1
  Saturation2/1 -> Scope1/3, Sum6/1  "Выход РТ"

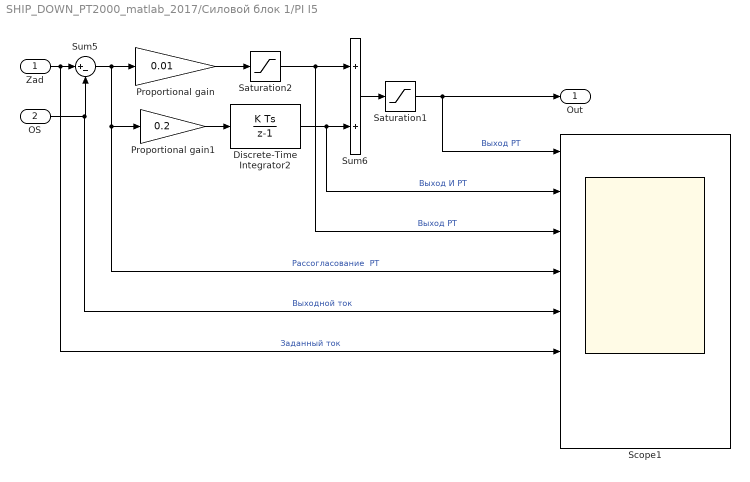
== system SHIP_DOWN_PT2000_matlab_2017/Силовой блок 1/PI I5 ==
  Zad : Inport
  OS : Inport  Port=2
  Discrete-Time Integrator2 : DiscreteIntegrator  SampleTime=-1  LimitOutput=on  UpperSaturationLimit=0.7  LowerSaturationLimit=0  ICPrevOutput=DiscIntNeverNeededParam  ICPrevScaledInput=DiscIntNeverNeededParam
  Proportional gain : Gain  Gain=0.01  SaturateOnIntegerOverflow=on  OutDataTypeStr=Inherit: Same as input  ParamDataTypeStr=Inherit: Same as input
  Proportional gain1 : Gain  Gain=0.2  SaturateOnIntegerOverflow=on  OutDataTypeStr=Inherit: Same as input  ParamDataTypeStr=Inherit: Same as input
  Saturation1 : Saturate  UpperLimit=0.7  LowerLimit=0
  Saturation2 : Saturate  UpperLimit=0.4  LowerLimit=0
  Scope1 : Scope  NumInputPorts=8
  Sum5 : Sum  Inputs=|+-  SaturateOnIntegerOverflow=on  InputSameDT=on  OutDataTypeStr=Inherit: Same as first input
  Sum6 : Sum  SaturateOnIntegerOverflow=on  InputSameDT=on  OutDataTypeStr=Inherit: Same as first input
  Out : Outport
  wires:
  Proportional gain/1 -> Saturation2/1
  Discrete-Time Integrator2/1 -> Sum6/2, Scope1/2  "Выход И РТ"
  OS/1 -> Scope1/5, Sum5/2  "Выходной ток"
  Zad/1 -> Scope1/6, Sum5/1  "Заданный ток"
  Sum5/1 -> Proportional gain1/1, Scope1/4, Proportional gain/1  "Рассогласование  РТ"
  Sum6/1 -> Saturation1/1
  Saturation1/1 -> Out/1, Scope1/1  "Выход РТ"
  Proportional gain1/1 -> Discrete-Time Integrator2/1
  Saturation2/1 -> Scope1/3, Sum6/1  "Выход РТ"

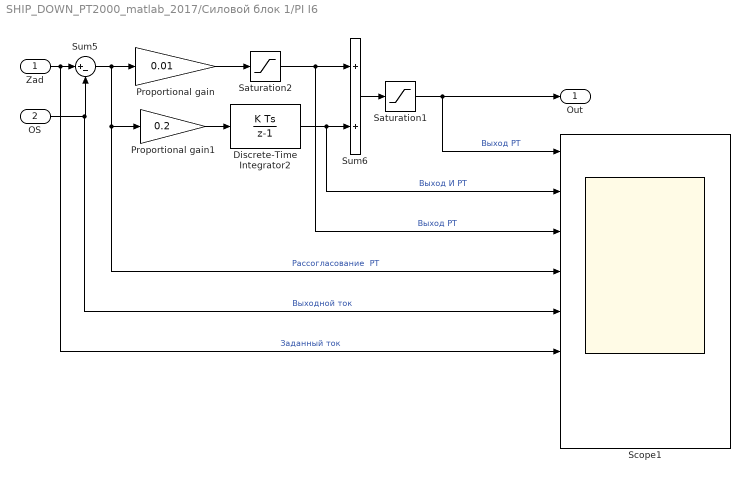
== system SHIP_DOWN_PT2000_matlab_2017/Силовой блок 1/PI I6 ==
  Zad : Inport
  OS : Inport  Port=2
  Discrete-Time Integrator2 : DiscreteIntegrator  SampleTime=-1  LimitOutput=on  UpperSaturationLimit=0.7  LowerSaturationLimit=0  ICPrevOutput=DiscIntNeverNeededParam  ICPrevScaledInput=DiscIntNeverNeededParam
  Proportional gain : Gain  Gain=0.01  SaturateOnIntegerOverflow=on  OutDataTypeStr=Inherit: Same as input  ParamDataTypeStr=Inherit: Same as input
  Proportional gain1 : Gain  Gain=0.2  SaturateOnIntegerOverflow=on  OutDataTypeStr=Inherit: Same as input  ParamDataTypeStr=Inherit: Same as input
  Saturation1 : Saturate  UpperLimit=0.7  LowerLimit=0
  Saturation2 : Saturate  UpperLimit=0.4  LowerLimit=0
  Scope1 : Scope  NumInputPorts=8
  Sum5 : Sum  Inputs=|+-  SaturateOnIntegerOverflow=on  InputSameDT=on  OutDataTypeStr=Inherit: Same as first input
  Sum6 : Sum  SaturateOnIntegerOverflow=on  InputSameDT=on  OutDataTypeStr=Inherit: Same as first input
  Out : Outport
  wires:
  Proportional gain/1 -> Saturation2/1
  Discrete-Time Integrator2/1 -> Sum6/2, Scope1/2  "Выход И РТ"
  OS/1 -> Scope1/5, Sum5/2  "Выходной ток"
  Zad/1 -> Scope1/6, Sum5/1  "Заданный ток"
  Sum5/1 -> Proportional gain1/1, Scope1/4, Proportional gain/1  "Рассогласование  РТ"
  Sum6/1 -> Saturation1/1
  Saturation1/1 -> Out/1, Scope1/1  "Выход РТ"
  Proportional gain1/1 -> Discrete-Time Integrator2/1
  Saturation2/1 -> Scope1/3, Sum6/1  "Выход РТ"

== system SHIP_DOWN_PT2000_matlab_2017/Силовой блок 1/PWM1 ==
  Uz : Inport
  Data Type Conversion : DataTypeConversion  OutDataTypeStr=boolean
  Delay1 : Delay  DelayLength=dellay_f1  InitialCondition=0  UseCircularBuffer=on
  Logical Operator : Logic  Operator=NOT  AllPortsSameDT=off  OutDataTypeStr=boolean
  Relay1 : Relay  OnSwitchValue=0.01  OffSwitchValue=-0.01
  Repeating Sequence1 : simulink/Sources/Repeating Sequence  rep_seq_t="[0  (1/(2*f)) (1/f)]"  rep_seq_y=[0 1 0]
  S-R Flip-Flop : simulink_extras/Flip Flops/S-R Flip-Flop  initial_condition=0
  Sum : Sum  Inputs=+-
  Terminator : Terminator
  CH1 : Outport
  wires:
  S-R Flip-Flop/1 -> CH1/1
  Data Type Conversion/1 -> S-R Flip-Flop/1
  Logical Operator/1 -> S-R Flip-Flop/2
  Relay1/1 -> Logical Operator/1, Data Type Conversion/1
  Uz/1 -> Sum/1
  Sum/1 -> Relay1/1
  S-R Flip-Flop/2 -> Terminator/1
  Repeating Sequence1/1 -> Delay1/1
  Delay1/1 -> Sum/2

== system SHIP_DOWN_PT2000_matlab_2017/Силовой блок 1/PWM2 ==
  Uz : Inport
  Data Type Conversion : DataTypeConversion  OutDataTypeStr=boolean
  Delay1 : Delay  DelayLength=dellay_f2  InitialCondition=0  UseCircularBuffer=on
  Logical Operator : Logic  Operator=NOT  AllPortsSameDT=off  OutDataTypeStr=boolean
  Relay1 : Relay  OnSwitchValue=0.01  OffSwitchValue=-0.01
  Repeating Sequence1 : simulink/Sources/Repeating Sequence  rep_seq_t="[0  (1/(2*f)) (1/f)]"  rep_seq_y=[0 1 0]
  S-R Flip-Flop : simulink_extras/Flip Flops/S-R Flip-Flop  initial_condition=0
  Sum : Sum  Inputs=+-
  Terminator : Terminator
  CH1 : Outport
  wires:
  S-R Flip-Flop/1 -> CH1/1
  Data Type Conversion/1 -> S-R Flip-Flop/1
  Logical Operator/1 -> S-R Flip-Flop/2
  Relay1/1 -> Logical Operator/1, Data Type Conversion/1
  Uz/1 -> Sum/1
  Sum/1 -> Relay1/1
  S-R Flip-Flop/2 -> Terminator/1
  Repeating Sequence1/1 -> Delay1/1
  Delay1/1 -> Sum/2

== system SHIP_DOWN_PT2000_matlab_2017/Силовой блок 1/PWM3 ==
  Uz : Inport
  Data Type Conversion : DataTypeConversion  OutDataTypeStr=boolean
  Delay1 : Delay  DelayLength=dellay_f3  InitialCondition=0  UseCircularBuffer=on
  Logical Operator : Logic  Operator=NOT  AllPortsSameDT=off  OutDataTypeStr=boolean
  Relay1 : Relay  OnSwitchValue=0.01  OffSwitchValue=-0.01
  Repeating Sequence1 : simulink/Sources/Repeating Sequence  rep_seq_t="[0  (1/(2*f)) (1/f)]"  rep_seq_y=[0 1 0]
  S-R Flip-Flop : simulink_extras/Flip Flops/S-R Flip-Flop  initial_condition=0
  Sum : Sum  Inputs=+-
  Terminator : Terminator
  CH1 : Outport
  wires:
  S-R Flip-Flop/1 -> CH1/1
  Data Type Conversion/1 -> S-R Flip-Flop/1
  Logical Operator/1 -> S-R Flip-Flop/2
  Relay1/1 -> Logical Operator/1, Data Type Conversion/1
  Uz/1 -> Sum/1
  Sum/1 -> Relay1/1
  S-R Flip-Flop/2 -> Terminator/1
  Repeating Sequence1/1 -> Delay1/1
  Delay1/1 -> Sum/2

== system SHIP_DOWN_PT2000_matlab_2017/Силовой блок 1/PWM4 ==
  Uz : Inport
  Data Type Conversion : DataTypeConversion  OutDataTypeStr=boolean
  Delay1 : Delay  DelayLength=dellay_f4  InitialCondition=0  UseCircularBuffer=on
  Logical Operator : Logic  Operator=NOT  AllPortsSameDT=off  OutDataTypeStr=boolean
  Relay1 : Relay  OnSwitchValue=0.01  OffSwitchValue=-0.01
  Repeating Sequence1 : simulink/Sources/Repeating Sequence  rep_seq_t="[0  (1/(2*f)) (1/f)]"  rep_seq_y=[0 1 0]
  S-R Flip-Flop : simulink_extras/Flip Flops/S-R Flip-Flop  initial_condition=0
  Sum : Sum  Inputs=+-
  Terminator : Terminator
  CH1 : Outport
  wires:
  S-R Flip-Flop/1 -> CH1/1
  Data Type Conversion/1 -> S-R Flip-Flop/1
  Logical Operator/1 -> S-R Flip-Flop/2
  Relay1/1 -> Logical Operator/1, Data Type Conversion/1
  Uz/1 -> Sum/1
  Sum/1 -> Relay1/1
  S-R Flip-Flop/2 -> Terminator/1
  Repeating Sequence1/1 -> Delay1/1
  Delay1/1 -> Sum/2

== system SHIP_DOWN_PT2000_matlab_2017/Силовой блок 1/PWM5 ==
  Uz : Inport
  Data Type Conversion : DataTypeConversion  OutDataTypeStr=boolean
  Delay1 : Delay  DelayLength=dellay_f5  InitialCondition=0  UseCircularBuffer=on
  Logical Operator : Logic  Operator=NOT  AllPortsSameDT=off  OutDataTypeStr=boolean
  Relay1 : Relay  OnSwitchValue=0.01  OffSwitchValue=-0.01
  Repeating Sequence1 : simulink/Sources/Repeating Sequence  rep_seq_t="[0  (1/(2*f)) (1/f)]"  rep_seq_y=[0 1 0]
  S-R Flip-Flop : simulink_extras/Flip Flops/S-R Flip-Flop  initial_condition=0
  Sum : Sum  Inputs=+-
  Terminator : Terminator
  CH1 : Outport
  wires:
  S-R Flip-Flop/1 -> CH1/1
  Data Type Conversion/1 -> S-R Flip-Flop/1
  Logical Operator/1 -> S-R Flip-Flop/2
  Relay1/1 -> Logical Operator/1, Data Type Conversion/1
  Uz/1 -> Sum/1
  Sum/1 -> Relay1/1
  S-R Flip-Flop/2 -> Terminator/1
  Repeating Sequence1/1 -> Delay1/1
  Delay1/1 -> Sum/2

== system SHIP_DOWN_PT2000_matlab_2017/Силовой блок 1/PWM6 ==
  Uz : Inport
  Data Type Conversion : DataTypeConversion  OutDataTypeStr=boolean
  Delay1 : Delay  DelayLength=dellay_f6  InitialCondition=0  UseCircularBuffer=on
  Logical Operator : Logic  Operator=NOT  AllPortsSameDT=off  OutDataTypeStr=boolean
  Relay1 : Relay  OnSwitchValue=0.01  OffSwitchValue=-0.01
  Repeating Sequence1 : simulink/Sources/Repeating Sequence  rep_seq_t="[0  (1/(2*f)) (1/f)]"  rep_seq_y=[0 1 0]
  S-R Flip-Flop : simulink_extras/Flip Flops/S-R Flip-Flop  initial_condition=0
  Sum : Sum  Inputs=+-
  Terminator : Terminator
  CH1 : Outport
  wires:
  S-R Flip-Flop/1 -> CH1/1
  Data Type Conversion/1 -> S-R Flip-Flop/1
  Logical Operator/1 -> S-R Flip-Flop/2
  Relay1/1 -> Logical Operator/1, Data Type Conversion/1
  Uz/1 -> Sum/1
  Sum/1 -> Relay1/1
  S-R Flip-Flop/2 -> Terminator/1
  Repeating Sequence1/1 -> Delay1/1
  Delay1/1 -> Sum/2

== system SHIP_DOWN_PT2000_matlab_2017/Силовой блок 2/PI I1 ==
  Zad : Inport
  OS : Inport  Port=2
  Discrete-Time Integrator2 : DiscreteIntegrator  SampleTime=-1  LimitOutput=on  UpperSaturationLimit=0.7  LowerSaturationLimit=0  ICPrevOutput=DiscIntNeverNeededParam  ICPrevScaledInput=DiscIntNeverNeededParam
  Proportional gain : Gain  Gain=0.01  SaturateOnIntegerOverflow=on  OutDataTypeStr=Inherit: Same as input  ParamDataTypeStr=Inherit: Same as input
  Proportional gain1 : Gain  Gain=0.2  SaturateOnIntegerOverflow=on  OutDataTypeStr=Inherit: Same as input  ParamDataTypeStr=Inherit: Same as input
  Saturation1 : Saturate  UpperLimit=0.7  LowerLimit=0
  Saturation2 : Saturate  UpperLimit=0.4  LowerLimit=0
  Scope1 : Scope  NumInputPorts=8
  Sum5 : Sum  Inputs=|+-  SaturateOnIntegerOverflow=on  InputSameDT=on  OutDataTypeStr=Inherit: Same as first input
  Sum6 : Sum  SaturateOnIntegerOverflow=on  InputSameDT=on  OutDataTypeStr=Inherit: Same as first input
  Out : Outport
  wires:
  Proportional gain/1 -> Saturation2/1
  Discrete-Time Integrator2/1 -> Sum6/2, Scope1/2  "Выход И РТ"
  OS/1 -> Scope1/5, Sum5/2  "Выходной ток"
  Zad/1 -> Scope1/6, Sum5/1  "Заданный ток"
  Sum5/1 -> Proportional gain1/1, Scope1/4, Proportional gain/1  "Рассогласование  РТ"
  Sum6/1 -> Saturation1/1
  Saturation1/1 -> Out/1, Scope1/1  "Выход РТ"
  Proportional gain1/1 -> Discrete-Time Integrator2/1
  Saturation2/1 -> Scope1/3, Sum6/1  "Выход РТ"

== system SHIP_DOWN_PT2000_matlab_2017/Силовой блок 2/PI I2 ==
  Zad : Inport
  OS : Inport  Port=2
  Discrete-Time Integrator2 : DiscreteIntegrator  SampleTime=-1  LimitOutput=on  UpperSaturationLimit=0.7  LowerSaturationLimit=0  ICPrevOutput=DiscIntNeverNeededParam  ICPrevScaledInput=DiscIntNeverNeededParam
  Proportional gain : Gain  Gain=0.01  SaturateOnIntegerOverflow=on  OutDataTypeStr=Inherit: Same as input  ParamDataTypeStr=Inherit: Same as input
  Proportional gain1 : Gain  Gain=0.2  SaturateOnIntegerOverflow=on  OutDataTypeStr=Inherit: Same as input  ParamDataTypeStr=Inherit: Same as input
  Saturation1 : Saturate  UpperLimit=0.7  LowerLimit=0
  Saturation2 : Saturate  UpperLimit=0.4  LowerLimit=0
  Scope1 : Scope  NumInputPorts=8
  Sum5 : Sum  Inputs=|+-  SaturateOnIntegerOverflow=on  InputSameDT=on  OutDataTypeStr=Inherit: Same as first input
  Sum6 : Sum  SaturateOnIntegerOverflow=on  InputSameDT=on  OutDataTypeStr=Inherit: Same as first input
  Out : Outport
  wires:
  Proportional gain/1 -> Saturation2/1
  Discrete-Time Integrator2/1 -> Sum6/2, Scope1/2  "Выход И РТ"
  OS/1 -> Scope1/5, Sum5/2  "Выходной ток"
  Zad/1 -> Scope1/6, Sum5/1  "Заданный ток"
  Sum5/1 -> Proportional gain1/1, Scope1/4, Proportional gain/1  "Рассогласование  РТ"
  Sum6/1 -> Saturation1/1
  Saturation1/1 -> Out/1, Scope1/1  "Выход РТ"
  Proportional gain1/1 -> Discrete-Time Integrator2/1
  Saturation2/1 -> Scope1/3, Sum6/1  "Выход РТ"

== system SHIP_DOWN_PT2000_matlab_2017/Силовой блок 2/PI I3 ==
  Zad : Inport
  OS : Inport  Port=2
  Discrete-Time Integrator2 : DiscreteIntegrator  SampleTime=-1  LimitOutput=on  UpperSaturationLimit=0.7  LowerSaturationLimit=0  ICPrevOutput=DiscIntNeverNeededParam  ICPrevScaledInput=DiscIntNeverNeededParam
  Proportional gain : Gain  Gain=0.01  SaturateOnIntegerOverflow=on  OutDataTypeStr=Inherit: Same as input  ParamDataTypeStr=Inherit: Same as input
  Proportional gain1 : Gain  Gain=0.2  SaturateOnIntegerOverflow=on  OutDataTypeStr=Inherit: Same as input  ParamDataTypeStr=Inherit: Same as input
  Saturation1 : Saturate  UpperLimit=0.7  LowerLimit=0
  Saturation2 : Saturate  UpperLimit=0.4  LowerLimit=0
  Scope1 : Scope  NumInputPorts=8
  Sum5 : Sum  Inputs=|+-  SaturateOnIntegerOverflow=on  InputSameDT=on  OutDataTypeStr=Inherit: Same as first input
  Sum6 : Sum  SaturateOnIntegerOverflow=on  InputSameDT=on  OutDataTypeStr=Inherit: Same as first input
  Out : Outport
  wires:
  Proportional gain/1 -> Saturation2/1
  Discrete-Time Integrator2/1 -> Sum6/2, Scope1/2  "Выход И РТ"
  OS/1 -> Scope1/5, Sum5/2  "Выходной ток"
  Zad/1 -> Scope1/6, Sum5/1  "Заданный ток"
  Sum5/1 -> Proportional gain1/1, Scope1/4, Proportional gain/1  "Рассогласование  РТ"
  Sum6/1 -> Saturation1/1
  Saturation1/1 -> Out/1, Scope1/1  "Выход РТ"
  Proportional gain1/1 -> Discrete-Time Integrator2/1
  Saturation2/1 -> Scope1/3, Sum6/1  "Выход РТ"

== system SHIP_DOWN_PT2000_matlab_2017/Силовой блок 2/PI I4 ==
  Zad : Inport
  OS : Inport  Port=2
  Discrete-Time Integrator2 : DiscreteIntegrator  SampleTime=-1  LimitOutput=on  UpperSaturationLimit=0.7  LowerSaturationLimit=0  ICPrevOutput=DiscIntNeverNeededParam  ICPrevScaledInput=DiscIntNeverNeededParam
  Proportional gain : Gain  Gain=0.01  SaturateOnIntegerOverflow=on  OutDataTypeStr=Inherit: Same as input  ParamDataTypeStr=Inherit: Same as input
  Proportional gain1 : Gain  Gain=0.2  SaturateOnIntegerOverflow=on  OutDataTypeStr=Inherit: Same as input  ParamDataTypeStr=Inherit: Same as input
  Saturation1 : Saturate  UpperLimit=0.7  LowerLimit=0
  Saturation2 : Saturate  UpperLimit=0.4  LowerLimit=0
  Scope1 : Scope  NumInputPorts=8
  Sum5 : Sum  Inputs=|+-  SaturateOnIntegerOverflow=on  InputSameDT=on  OutDataTypeStr=Inherit: Same as first input
  Sum6 : Sum  SaturateOnIntegerOverflow=on  InputSameDT=on  OutDataTypeStr=Inherit: Same as first input
  Out : Outport
  wires:
  Proportional gain/1 -> Saturation2/1
  Discrete-Time Integrator2/1 -> Sum6/2, Scope1/2  "Выход И РТ"
  OS/1 -> Scope1/5, Sum5/2  "Выходной ток"
  Zad/1 -> Scope1/6, Sum5/1  "Заданный ток"
  Sum5/1 -> Proportional gain1/1, Scope1/4, Proportional gain/1  "Рассогласование  РТ"
  Sum6/1 -> Saturation1/1
  Saturation1/1 -> Out/1, Scope1/1  "Выход РТ"
  Proportional gain1/1 -> Discrete-Time Integrator2/1
  Saturation2/1 -> Scope1/3, Sum6/1  "Выход РТ"

== system SHIP_DOWN_PT2000_matlab_2017/Силовой блок 2/PI I5 ==
  Zad : Inport
  OS : Inport  Port=2
  Discrete-Time Integrator2 : DiscreteIntegrator  SampleTime=-1  LimitOutput=on  UpperSaturationLimit=0.7  LowerSaturationLimit=0  ICPrevOutput=DiscIntNeverNeededParam  ICPrevScaledInput=DiscIntNeverNeededParam
  Proportional gain : Gain  Gain=0.01  SaturateOnIntegerOverflow=on  OutDataTypeStr=Inherit: Same as input  ParamDataTypeStr=Inherit: Same as input
  Proportional gain1 : Gain  Gain=0.2  SaturateOnIntegerOverflow=on  OutDataTypeStr=Inherit: Same as input  ParamDataTypeStr=Inherit: Same as input
  Saturation1 : Saturate  UpperLimit=0.7  LowerLimit=0
  Saturation2 : Saturate  UpperLimit=0.4  LowerLimit=0
  Scope1 : Scope  NumInputPorts=8
  Sum5 : Sum  Inputs=|+-  SaturateOnIntegerOverflow=on  InputSameDT=on  OutDataTypeStr=Inherit: Same as first input
  Sum6 : Sum  SaturateOnIntegerOverflow=on  InputSameDT=on  OutDataTypeStr=Inherit: Same as first input
  Out : Outport
  wires:
  Proportional gain/1 -> Saturation2/1
  Discrete-Time Integrator2/1 -> Sum6/2, Scope1/2  "Выход И РТ"
  OS/1 -> Scope1/5, Sum5/2  "Выходной ток"
  Zad/1 -> Scope1/6, Sum5/1  "Заданный ток"
  Sum5/1 -> Proportional gain1/1, Scope1/4, Proportional gain/1  "Рассогласование  РТ"
  Sum6/1 -> Saturation1/1
  Saturation1/1 -> Out/1, Scope1/1  "Выход РТ"
  Proportional gain1/1 -> Discrete-Time Integrator2/1
  Saturation2/1 -> Scope1/3, Sum6/1  "Выход РТ"

== system SHIP_DOWN_PT2000_matlab_2017/Силовой блок 2/PI I6 ==
  Zad : Inport
  OS : Inport  Port=2
  Discrete-Time Integrator2 : DiscreteIntegrator  SampleTime=-1  LimitOutput=on  UpperSaturationLimit=0.7  LowerSaturationLimit=0  ICPrevOutput=DiscIntNeverNeededParam  ICPrevScaledInput=DiscIntNeverNeededParam
  Proportional gain : Gain  Gain=0.01  SaturateOnIntegerOverflow=on  OutDataTypeStr=Inherit: Same as input  ParamDataTypeStr=Inherit: Same as input
  Proportional gain1 : Gain  Gain=0.2  SaturateOnIntegerOverflow=on  OutDataTypeStr=Inherit: Same as input  ParamDataTypeStr=Inherit: Same as input
  Saturation1 : Saturate  UpperLimit=0.7  LowerLimit=0
  Saturation2 : Saturate  UpperLimit=0.4  LowerLimit=0
  Scope1 : Scope  NumInputPorts=8
  Sum5 : Sum  Inputs=|+-  SaturateOnIntegerOverflow=on  InputSameDT=on  OutDataTypeStr=Inherit: Same as first input
  Sum6 : Sum  SaturateOnIntegerOverflow=on  InputSameDT=on  OutDataTypeStr=Inherit: Same as first input
  Out : Outport
  wires:
  Proportional gain/1 -> Saturation2/1
  Discrete-Time Integrator2/1 -> Sum6/2, Scope1/2  "Выход И РТ"
  OS/1 -> Scope1/5, Sum5/2  "Выходной ток"
  Zad/1 -> Scope1/6, Sum5/1  "Заданный ток"
  Sum5/1 -> Proportional gain1/1, Scope1/4, Proportional gain/1  "Рассогласование  РТ"
  Sum6/1 -> Saturation1/1
  Saturation1/1 -> Out/1, Scope1/1  "Выход РТ"
  Proportional gain1/1 -> Discrete-Time Integrator2/1
  Saturation2/1 -> Scope1/3, Sum6/1  "Выход РТ"

== system SHIP_DOWN_PT2000_matlab_2017/Силовой блок 2/PWM1 ==
  Uz : Inport
  Data Type Conversion : DataTypeConversion  OutDataTypeStr=boolean
  Delay1 : Delay  DelayLength=dellay_f1  InitialCondition=0  UseCircularBuffer=on
  Logical Operator : Logic  Operator=NOT  AllPortsSameDT=off  OutDataTypeStr=boolean
  Relay1 : Relay  OnSwitchValue=0.01  OffSwitchValue=-0.01
  Repeating Sequence1 : simulink/Sources/Repeating Sequence  rep_seq_t="[0  (1/(2*f)) (1/f)]"  rep_seq_y=[0 1 0]
  S-R Flip-Flop : simulink_extras/Flip Flops/S-R Flip-Flop  initial_condition=0
  Sum : Sum  Inputs=+-
  Terminator : Terminator
  CH1 : Outport
  wires:
  S-R Flip-Flop/1 -> CH1/1
  Data Type Conversion/1 -> S-R Flip-Flop/1
  Logical Operator/1 -> S-R Flip-Flop/2
  Relay1/1 -> Logical Operator/1, Data Type Conversion/1
  Uz/1 -> Sum/1
  Sum/1 -> Relay1/1
  S-R Flip-Flop/2 -> Terminator/1
  Repeating Sequence1/1 -> Delay1/1
  Delay1/1 -> Sum/2

== system SHIP_DOWN_PT2000_matlab_2017/Силовой блок 2/PWM2 ==
  Uz : Inport
  Data Type Conversion : DataTypeConversion  OutDataTypeStr=boolean
  Delay1 : Delay  DelayLength=dellay_f2  InitialCondition=0  UseCircularBuffer=on
  Logical Operator : Logic  Operator=NOT  AllPortsSameDT=off  OutDataTypeStr=boolean
  Relay1 : Relay  OnSwitchValue=0.01  OffSwitchValue=-0.01
  Repeating Sequence1 : simulink/Sources/Repeating Sequence  rep_seq_t="[0  (1/(2*f)) (1/f)]"  rep_seq_y=[0 1 0]
  S-R Flip-Flop : simulink_extras/Flip Flops/S-R Flip-Flop  initial_condition=0
  Sum : Sum  Inputs=+-
  Terminator : Terminator
  CH1 : Outport
  wires:
  S-R Flip-Flop/1 -> CH1/1
  Data Type Conversion/1 -> S-R Flip-Flop/1
  Logical Operator/1 -> S-R Flip-Flop/2
  Relay1/1 -> Logical Operator/1, Data Type Conversion/1
  Uz/1 -> Sum/1
  Sum/1 -> Relay1/1
  S-R Flip-Flop/2 -> Terminator/1
  Repeating Sequence1/1 -> Delay1/1
  Delay1/1 -> Sum/2

== system SHIP_DOWN_PT2000_matlab_2017/Силовой блок 2/PWM3 ==
  Uz : Inport
  Data Type Conversion : DataTypeConversion  OutDataTypeStr=boolean
  Delay1 : Delay  DelayLength=dellay_f3  InitialCondition=0  UseCircularBuffer=on
  Logical Operator : Logic  Operator=NOT  AllPortsSameDT=off  OutDataTypeStr=boolean
  Relay1 : Relay  OnSwitchValue=0.01  OffSwitchValue=-0.01
  Repeating Sequence1 : simulink/Sources/Repeating Sequence  rep_seq_t="[0  (1/(2*f)) (1/f)]"  rep_seq_y=[0 1 0]
  S-R Flip-Flop : simulink_extras/Flip Flops/S-R Flip-Flop  initial_condition=0
  Sum : Sum  Inputs=+-
  Terminator : Terminator
  CH1 : Outport
  wires:
  S-R Flip-Flop/1 -> CH1/1
  Data Type Conversion/1 -> S-R Flip-Flop/1
  Logical Operator/1 -> S-R Flip-Flop/2
  Relay1/1 -> Logical Operator/1, Data Type Conversion/1
  Uz/1 -> Sum/1
  Sum/1 -> Relay1/1
  S-R Flip-Flop/2 -> Terminator/1
  Repeating Sequence1/1 -> Delay1/1
  Delay1/1 -> Sum/2
